simulink model "model"  (R2023b)
settings: Solver=VariableStepAuto  StartTime=0.0  StopTime=10.0  RelTol=1e-3
undefined symbols (not defined in the file): DiscIntNeverNeededParam, fd74c4e2, magnitude, Newton, Raphson
libraries: simulink x102, slpidlib x35
(part 3 of 5)

== system model/cfblk53/cfblk10 ==
  cfblk1 : Inport
  cfblk10 : Inport  Port=2
  cfblk11 : Delay  SampleTime=1
  cfblk3 : simulink/Discrete/Tapped Delay  vinit=0.0  samptime=-1  NumDelays=1  DelayOrder=Oldest  includeCurrent=off
  cfblk4 : slpidlib/PID Controller  Controller=PID  Form=Parallel  TimeDomain=Discrete-time  UseExternalTs=off  SampleTime=1  IntegratorMethod=Forward Euler  FilterMethod=Forward Euler  ControllerParametersSource=internal  P=1  I=1  UseKiTs=off  D=0  N=100  UseFilter=on  TunerSelectOption=Transfer Function Based (PID Tuner App)  InitialConditionSource=internal  InitialConditionForIntegrator=0  InitialConditionForFilter=0  DifferentiatorICPrevScaledInput=0  ExternalReset=none  TrackingMode=off  Kt=1  LimitOutput=off  SatLimitsSource=internal  UpperSaturationLimit=inf  LowerSaturationLimit=-inf  LinearizeAsGain=off  AntiWindupMode=none  Kb=1  LimitIntegrator=off  UpperIntegratorSaturationLimit=inf  LowerIntegratorSaturationLimit=-inf  POutMin=[]  POutMax=[]  IOutMin=[]  IOutMax=[]  DOutMin=[]  DOutMax=[]  NOutMin=[]  NOutMax=[]  SumOutMin=[]  SumOutMax=[]  SaturationOutMin=[]  SaturationOutMax=[]  PParamMin=[]  PParamMax=[]  IParamMin=[]  IParamMax=[]  DParamMin=[]  DParamMax=[]  NParamMin=[]  NParamMax=[]  KbParamMin=[]  KbParamMax=[]  KtParamMin=[]  KtParamMax=[]  KbOutMin=[]  KbOutMax=[]  KtOutMin=[]  KtOutMax=[]  IntegratorOutMin=[]  IntegratorOutMax=[]  FilterOutMin=[]  FilterOutMax=[]  SumI1OutMin=[]  SumI1OutMax=[]  SumI2OutMin=[]  SumI2OutMax=[]  SumI3OutMin=[]  SumI3OutMax=[]  SumI4OutMin=[]  SumI4OutMax=[]  SumDOutMin=[]  SumDOutMax=[]  DifferentiatorOutMin=[]  DifferentiatorOutMax=[]  FilterDiffOutCoefMin=[]  FilterDiffOutCoefMax=[]  ReciprocalOutMin=[]  ReciprocalOutMax=[]  SumDenOutMin=[]  SumDenOutMax=[]  SumNumOutMin=[]  SumNumOutMax=[]  DivideOutMin=[]  DivideOutMax=[]  UdiffTsProdOutMin=[]  UdiffTsProdOutMax=[]  NTsProdOutMin=[]  NTsProdOutMax=[]  UintegralTsProdOutMin=[]  UintegralTsProdOutMax=[]  UngainTsProdOutMin=[]  UngainTsProdOutMax=[]  ClampingZeroOutDataTypeStr=Inherit: Inherit via back propagation  ClampingZeroOutMin=[]  ClampingZeroOutMax=[]  FilterDenConstantOutDataTypeStr=Inherit: Inherit via back propagation  FilterDenConstantOutMin=[]  FilterDenConstantOutMax=[]  PCopyOutDataTypeStr=Inherit: Inherit via back propagation  PCopyOutMin=[]  PCopyOutMax=[]  NCopyOutDataTypeStr=Inherit: Inherit via back propagation  NCopyOutMin=[]  NCopyOutMax=[]  IntegratorContinuousStateAttributes=''  IntegratorStateMustResolveToSignalObject=off  IntegratorRTWStateStorageClass=Auto  FilterContinuousStateAttributes=''  FilterStateMustResolveToSignalObject=off  FilterRTWStateStorageClass=Auto  ParallelPVariant=InternalParameters  IdealPVariant=Disabled  IVariant=InternalParameters  DVariant=InternalParameters  IntegratorVariant=Discrete  SatVariant=Disabled  AWVariant=Passthrough  PCopyVariant=Disabled  TRVariant=Disabled  FdbkBlocksVariant=Forward  IdealPFdbkVariant=Disabled  SatFdbkVariant=Disabled  DerivativeFilterVariant=ForwardEulerFilter  NVariant=InternalParameters  NCopyVariant=Disabled  FilterICVariant=InternalICsFilter  IntegratorICVariant=InternalICs  ExternalResetVariant=Disabled  TRSumVariant=Passthrough  SumFdbkVariant=Disabled  SumVariant=Sum_PID  TsampFilterVariant=InternalTs  TsampNgainVariant=Passthrough  TsampIntegralVariant=Disabled_SignalSpec  ExternalSaturationOutDataTypeStr=Inherit: Same as second input
      settings: LibrarySourceBlock=simulink/Discrete/Discrete PID Controller
  cfblk5 : DiscreteIntegrator  ICPrevOutput=DiscIntNeverNeededParam  ICPrevScaledInput=DiscIntNeverNeededParam
  cfblk6 : Reshape
  cfblk7 : Sum  Inputs=+-
  cfblk8 : Gain  Gain=[817664659.316137]
  cfblk9 : ComplexToMagnitudeAngle
  cfblk2 : Outport
  wires:
  cfblk7/1 -> cfblk2/1
  cfblk1/1 -> cfblk7/1
  cfblk4/1 -> cfblk6/1
  cfblk8/1 -> cfblk9/1
  cfblk9/1 -> cfblk3/1
  cfblk3/1 -> cfblk5/1
  cfblk10/1 -> cfblk8/1
  cfblk9/2 -> cfblk7/2
  cfblk6/1 -> cfblk11/1
  cfblk11/1 -> cfblk4/1

== system model/cfblk53/cfblk11 ==
  cfblk1 : Inport
  cfblk7 : Inport  Port=2
  cfblk8 : Inport  Port=3
  cfblk9 : Inport  Port=4
  cfblk3 : simulink/Discrete/Transfer Fcn Lead or Lag  PoleZ=0.95  ZeroZ=0.75  ICPrevOutput=0.0  ICPrevInput=0.0  DoSatur=off
  cfblk4 : simulink/Discrete/Difference  ICPrevInput=0.0  OutMin=[]  OutMax=[]  OutDataTypeStr=Inherit: Inherit via back propagation  OutDataType=fixdt(1, 16)  OutScaling=2^-10  DoSatur=off
  cfblk5 : Product  Inputs=*
  cfblk6 : Sum  Inputs=+
  cfblk2 : Outport
  cfblk10 : Outport  Port=2
  cfblk11 : Outport  Port=3
  wires:
  cfblk5/1 -> cfblk2/1
  cfblk3/1 -> cfblk10/1
  cfblk6/1 -> cfblk11/1
  cfblk1/1 -> cfblk3/1
  cfblk8/1 -> cfblk6/1
  cfblk4/1 -> cfblk5/1
  cfblk7/1 -> cfblk4/1

== system model/cfblk53/cfblk12 ==
  cfblk1 : Inport
  cfblk13 : Inport  Port=2
  cfblk14 : Inport  Port=3
  cfblk10 : Constant  Value=[-206110537.418355]  SampleTime=1
  cfblk11 : Constant  Value=[146359783.021186]  SampleTime=1
  cfblk12 : Constant  Value=[-708907228.749983]  SampleTime=1
  cfblk3 : DiscreteZeroPole  Poles=[0 0.5]  Gain=1
  cfblk4 : DiscreteFilter  SampleTime=1
  cfblk5 : Delay  DelayLengthSource=Input port  SampleTime=1
      settings: InputPortMap=u0,p1
  cfblk6 : DiscreteStateSpace
  cfblk7 : Abs  SaturateOnIntegerOverflow=off
  cfblk8 : Product
  cfblk9 : Sin  TimeSource=Use external signal  SampleTime=0
  cfblk2 : Outport
  wires:
  cfblk3/1 -> cfblk6/1
  cfblk10/1 -> cfblk4/1
  cfblk7/1 -> cfblk8/1
  cfblk12/1 -> cfblk8/2
  cfblk9/1 -> cfblk2/1
  cfblk6/1 -> cfblk9/1
  cfblk8/1 -> cfblk5/1
  cfblk13/1 -> cfblk3/1
  cfblk1/1 -> cfblk7/1
  cfblk14/1 -> cfblk5/2

== system model/cfblk55/cfblk10 ==
  cfblk1 : Inport
  cfblk12 : Inport  Port=2
  cfblk13 : Inport  Port=3
  cfblk14 : Inport  Port=4
  cfblk10 : Constant  Value=[62866536.244015]  SampleTime=1
  cfblk11 : Constant  Value=[-503289504.904032]  SampleTime=1
  cfblk3 : slpidlib/PID Controller (2DOF)  Controller=PID  Form=Parallel  TimeDomain=Discrete-time  UseExternalTs=off  SampleTime=1  IntegratorMethod=Forward Euler  FilterMethod=Forward Euler  ControllerParametersSource=internal  P=1  I=1  UseKiTs=off  D=0  N=100  UseFilter=on  b=1  c=1  TunerSelectOption=Transfer Function Based (PID Tuner App)  InitialConditionSource=internal  InitialConditionForIntegrator=0  InitialConditionForFilter=0  DifferentiatorICPrevScaledInput=0  ExternalReset=none  TrackingMode=off  Kt=1  LimitOutput=off  SatLimitsSource=internal  UpperSaturationLimit=inf  LowerSaturationLimit=-inf  LinearizeAsGain=off  AntiWindupMode=none  Kb=1  LimitIntegrator=off  UpperIntegratorSaturationLimit=inf  LowerIntegratorSaturationLimit=-inf  POutMin=[]  POutMax=[]  IOutMin=[]  IOutMax=[]  DOutMin=[]  DOutMax=[]  NOutMin=[]  NOutMax=[]  bOutMin=[]  bOutMax=[]  cOutMin=[]  cOutMax=[]  SumOutMin=[]  SumOutMax=[]  SaturationOutMin=[]  SaturationOutMax=[]  PParamMin=[]  PParamMax=[]  IParamMin=[]  IParamMax=[]  DParamMin=[]  DParamMax=[]  NParamMin=[]  NParamMax=[]  bParamMin=[]  bParamMax=[]  cParamMin=[]  cParamMax=[]  KbParamMin=[]  KbParamMax=[]  KtParamMin=[]  KtParamMax=[]  KbOutMin=[]  KbOutMax=[]  KtOutMin=[]  KtOutMax=[]  IntegratorOutMin=[]  IntegratorOutMax=[]  FilterOutMin=[]  FilterOutMax=[]  SumI1OutMin=[]  SumI1OutMax=[]  SumI2OutMin=[]  SumI2OutMax=[]  SumI3OutMin=[]  SumI3OutMax=[]  SumI4OutMin=[]  SumI4OutMax=[]  SumDOutMin=[]  SumDOutMax=[]  Sum1OutMin=[]  Sum1OutMax=[]  Sum2OutMin=[]  Sum2OutMax=[]  Sum3OutMin=[]  Sum3OutMax=[]  DifferentiatorOutMin=[]  DifferentiatorOutMax=[]  FilterDiffOutCoefMin=[]  FilterDiffOutCoefMax=[]  ReciprocalOutMin=[]  ReciprocalOutMax=[]  SumDenOutMin=[]  SumDenOutMax=[]  SumNumOutMin=[]  SumNumOutMax=[]  DivideOutMin=[]  DivideOutMax=[]  UdiffTsProdOutMin=[]  UdiffTsProdOutMax=[]  NTsProdOutMin=[]  NTsProdOutMax=[]  UintegralTsProdOutMin=[]  UintegralTsProdOutMax=[]  UngainTsProdOutMin=[]  UngainTsProdOutMax=[]  ClampingZeroOutDataTypeStr=Inherit: Inherit via back propagation  ClampingZeroOutMin=[]  ClampingZeroOutMax=[]  FilterDenConstantOutDataTypeStr=Inherit: Inherit via back propagation  FilterDenConstantOutMin=[]  FilterDenConstantOutMax=[]  PCopyOutDataTypeStr=Inherit: Inherit via back propagation  PCopyOutMin=[]  PCopyOutMax=[]  NCopyOutDataTypeStr=Inherit: Inherit via back propagation  NCopyOutMin=[]  NCopyOutMax=[]  IntegratorContinuousStateAttributes=''  IntegratorStateMustResolveToSignalObject=off  IntegratorRTWStateStorageClass=Auto  FilterContinuousStateAttributes=''  FilterStateMustResolveToSignalObject=off  FilterRTWStateStorageClass=Auto  ParallelPVariant=InternalParameters  IdealPVariant=Disabled  IVariant=InternalParameters  DVariant=InternalParameters  bVariant=InternalParameters  cVariant=InternalParameters  IntegratorVariant=Discrete  SatVariant=Disabled  AWVariant=Passthrough  PCopyVariant=Disabled  TRVariant=Disabled  FdbkBlocksVariant=Forward  IdealPFdbkVariant=Disabled  SatFdbkVariant=Disabled  DerivativeFilterVariant=ForwardEulerFilter  NVariant=InternalParameters  NCopyVariant=Disabled  FilterICVariant=InternalICsFilter  IntegratorICVariant=InternalICs  ExternalResetVariant=Disabled  TRSumVariant=Passthrough  SumFdbkVariant=Disabled  SumVariant=Sum_PID  TsampFilterVariant=InternalTs  TsampNgainVariant=Passthrough  TsampIntegralVariant=Disabled_SignalSpec  ExternalSaturationOutDataTypeStr=Inherit: Same as second input
      settings: LibrarySourceBlock=simulink/Discrete/Discrete PID Controller (2DOF)
  cfblk4 : slpidlib/PID Controller (2DOF)  Controller=PID  Form=Parallel  TimeDomain=Discrete-time  UseExternalTs=off  SampleTime=1  IntegratorMethod=Forward Euler  FilterMethod=Forward Euler  ControllerParametersSource=internal  P=1  I=1  UseKiTs=off  D=0  N=100  UseFilter=on  b=1  c=1  TunerSelectOption=Transfer Function Based (PID Tuner App)  InitialConditionSource=internal  InitialConditionForIntegrator=0  InitialConditionForFilter=0  DifferentiatorICPrevScaledInput=0  ExternalReset=none  TrackingMode=off  Kt=1  LimitOutput=off  SatLimitsSource=internal  UpperSaturationLimit=inf  LowerSaturationLimit=-inf  LinearizeAsGain=off  AntiWindupMode=none  Kb=1  LimitIntegrator=off  UpperIntegratorSaturationLimit=inf  LowerIntegratorSaturationLimit=-inf  POutMin=[]  POutMax=[]  IOutMin=[]  IOutMax=[]  DOutMin=[]  DOutMax=[]  NOutMin=[]  NOutMax=[]  bOutMin=[]  bOutMax=[]  cOutMin=[]  cOutMax=[]  SumOutMin=[]  SumOutMax=[]  SaturationOutMin=[]  SaturationOutMax=[]  PParamMin=[]  PParamMax=[]  IParamMin=[]  IParamMax=[]  DParamMin=[]  DParamMax=[]  NParamMin=[]  NParamMax=[]  bParamMin=[]  bParamMax=[]  cParamMin=[]  cParamMax=[]  KbParamMin=[]  KbParamMax=[]  KtParamMin=[]  KtParamMax=[]  KbOutMin=[]  KbOutMax=[]  KtOutMin=[]  KtOutMax=[]  IntegratorOutMin=[]  IntegratorOutMax=[]  FilterOutMin=[]  FilterOutMax=[]  SumI1OutMin=[]  SumI1OutMax=[]  SumI2OutMin=[]  SumI2OutMax=[]  SumI3OutMin=[]  SumI3OutMax=[]  SumI4OutMin=[]  SumI4OutMax=[]  SumDOutMin=[]  SumDOutMax=[]  Sum1OutMin=[]  Sum1OutMax=[]  Sum2OutMin=[]  Sum2OutMax=[]  Sum3OutMin=[]  Sum3OutMax=[]  DifferentiatorOutMin=[]  DifferentiatorOutMax=[]  FilterDiffOutCoefMin=[]  FilterDiffOutCoefMax=[]  ReciprocalOutMin=[]  ReciprocalOutMax=[]  SumDenOutMin=[]  SumDenOutMax=[]  SumNumOutMin=[]  SumNumOutMax=[]  DivideOutMin=[]  DivideOutMax=[]  UdiffTsProdOutMin=[]  UdiffTsProdOutMax=[]  NTsProdOutMin=[]  NTsProdOutMax=[]  UintegralTsProdOutMin=[]  UintegralTsProdOutMax=[]  UngainTsProdOutMin=[]  UngainTsProdOutMax=[]  ClampingZeroOutDataTypeStr=Inherit: Inherit via back propagation  ClampingZeroOutMin=[]  ClampingZeroOutMax=[]  FilterDenConstantOutDataTypeStr=Inherit: Inherit via back propagation  FilterDenConstantOutMin=[]  FilterDenConstantOutMax=[]  PCopyOutDataTypeStr=Inherit: Inherit via back propagation  PCopyOutMin=[]  PCopyOutMax=[]  NCopyOutDataTypeStr=Inherit: Inherit via back propagation  NCopyOutMin=[]  NCopyOutMax=[]  IntegratorContinuousStateAttributes=''  IntegratorStateMustResolveToSignalObject=off  IntegratorRTWStateStorageClass=Auto  FilterContinuousStateAttributes=''  FilterStateMustResolveToSignalObject=off  FilterRTWStateStorageClass=Auto  ParallelPVariant=InternalParameters  IdealPVariant=Disabled  IVariant=InternalParameters  DVariant=InternalParameters  bVariant=InternalParameters  cVariant=InternalParameters  IntegratorVariant=Discrete  SatVariant=Disabled  AWVariant=Passthrough  PCopyVariant=Disabled  TRVariant=Disabled  FdbkBlocksVariant=Forward  IdealPFdbkVariant=Disabled  SatFdbkVariant=Disabled  DerivativeFilterVariant=ForwardEulerFilter  NVariant=InternalParameters  NCopyVariant=Disabled  FilterICVariant=InternalICsFilter  IntegratorICVariant=InternalICs  ExternalResetVariant=Disabled  TRSumVariant=Passthrough  SumFdbkVariant=Disabled  SumVariant=Sum_PID  TsampFilterVariant=InternalTs  TsampNgainVariant=Passthrough  TsampIntegralVariant=Disabled_SignalSpec  ExternalSaturationOutDataTypeStr=Inherit: Same as second input
      settings: LibrarySourceBlock=simulink/Discrete/Discrete PID Controller (2DOF)
  cfblk5 : DiscreteStateSpace
  cfblk6 : Bias  Bias=[716171832.572191]  SaturateOnIntegerOverflow=off
  cfblk7 : Polyval  Coefs=[ +2.081618890e-019, -1.441693666e-014, +4.719686976e-010, -8.536869453e-006, +1.621573104e-001, -8.087801117e+001 ]
  cfblk8 : Constant  Value=[-316048415.208695]  SampleTime=1
  cfblk9 : Constant  Value=[-244945707.494813]  SampleTime=1
  cfblk2 : Outport
  cfblk15 : Outport  Port=2
  wires:
  cfblk6/1 -> cfblk5/1
  cfblk5/1 -> cfblk3/1
  cfblk1/1 -> cfblk4/1
  cfblk9/1 -> cfblk4/2
  cfblk8/1 -> cfblk3/2
  cfblk3/1 -> cfblk7/1
  cfblk10/1 -> cfblk15/1
  cfblk12/1 -> cfblk2/1
  cfblk13/1 -> cfblk6/1

== system model/cfblk55/cfblk11 ==
  cfblk1 : Inport
  cfblk9 : Inport  Port=2
  cfblk10 : Inport  Port=3
  cfblk11 : Inport  Port=4
  cfblk12 : Inport  Port=5
  cfblk13 : Inport  Port=6
  cfblk3 : DiscreteIntegrator  ICPrevOutput=DiscIntNeverNeededParam  ICPrevScaledInput=DiscIntNeverNeededParam
  cfblk4 : DiscreteStateSpace
  cfblk5 : ComplexToRealImag
  cfblk6 : Sum  Inputs=+-
  cfblk7 : Constant  Value=[-907148050.764415]  SampleTime=1
  cfblk8 : Constant  Value=[-534592741.405864]  SampleTime=1
  cfblk2 : Outport
  cfblk14 : Outport  Port=2
  wires:
  cfblk3/1 -> cfblk5/1
  cfblk1/1 -> cfblk14/1
  cfblk6/1 -> cfblk2/1
  cfblk8/1 -> cfblk6/1
  cfblk12/1 -> cfblk3/1
  cfblk11/1 -> cfblk4/1
  cfblk10/1 -> cfblk6/2

== system model/cfblk55/cfblk12 ==
  cfblk1 : Inport
  cfblk10 : Inport  Port=2
  cfblk11 : Inport  Port=3
  cfblk3 : simulink/Discrete/Transfer Fcn First Order  PoleZ=0.95  ICPrevOutput=0.0  DoSatur=off
  cfblk4 : UnitDelay  HasFrameUpgradeWarning=on
  cfblk5 : DiscreteFilter  SampleTime=1
  cfblk6 : simulink/Discrete/Difference  ICPrevInput=0.0  OutMin=[]  OutMax=[]  OutDataTypeStr=Inherit: Inherit via back propagation  OutDataType=fixdt(1, 16)  OutScaling=2^-10  DoSatur=off
  cfblk7 : Sqrt  Operator=rSqrt  AlgorithmType=Newton-Raphson
  cfblk8 : Product  Inputs=*
  cfblk9 : Constant  Value=[-99960536.236063]  SampleTime=1
  cfblk2 : Outport
  cfblk12 : Outport  Port=2
  wires:
  cfblk11/1 -> cfblk8/1
  cfblk9/1 -> cfblk3/1
  cfblk1/1 -> cfblk12/1
  cfblk8/1 -> cfblk5/1
  cfblk10/1 -> cfblk6/1
  cfblk6/1 -> cfblk4/1
  cfblk5/1 -> cfblk2/1
  cfblk4/1 -> cfblk7/1

== system model/cfblk56/cfblk10 ==
  cfblk1 : Inport
  cfblk7 : Inport  Port=2
  cfblk8 : Inport  Port=3
  cfblk3 : slpidlib/PID Controller (2DOF)  Controller=PID  Form=Parallel  TimeDomain=Discrete-time  UseExternalTs=off  SampleTime=1  IntegratorMethod=Forward Euler  FilterMethod=Forward Euler  ControllerParametersSource=internal  P=1  I=1  UseKiTs=off  D=0  N=100  UseFilter=on  b=1  c=1  TunerSelectOption=Transfer Function Based (PID Tuner App)  InitialConditionSource=internal  InitialConditionForIntegrator=0  InitialConditionForFilter=0  DifferentiatorICPrevScaledInput=0  ExternalReset=none  TrackingMode=off  Kt=1  LimitOutput=off  SatLimitsSource=internal  UpperSaturationLimit=inf  LowerSaturationLimit=-inf  LinearizeAsGain=off  AntiWindupMode=none  Kb=1  LimitIntegrator=off  UpperIntegratorSaturationLimit=inf  LowerIntegratorSaturationLimit=-inf  POutMin=[]  POutMax=[]  IOutMin=[]  IOutMax=[]  DOutMin=[]  DOutMax=[]  NOutMin=[]  NOutMax=[]  bOutMin=[]  bOutMax=[]  cOutMin=[]  cOutMax=[]  SumOutMin=[]  SumOutMax=[]  SaturationOutMin=[]  SaturationOutMax=[]  PParamMin=[]  PParamMax=[]  IParamMin=[]  IParamMax=[]  DParamMin=[]  DParamMax=[]  NParamMin=[]  NParamMax=[]  bParamMin=[]  bParamMax=[]  cParamMin=[]  cParamMax=[]  KbParamMin=[]  KbParamMax=[]  KtParamMin=[]  KtParamMax=[]  KbOutMin=[]  KbOutMax=[]  KtOutMin=[]  KtOutMax=[]  IntegratorOutMin=[]  IntegratorOutMax=[]  FilterOutMin=[]  FilterOutMax=[]  SumI1OutMin=[]  SumI1OutMax=[]  SumI2OutMin=[]  SumI2OutMax=[]  SumI3OutMin=[]  SumI3OutMax=[]  SumI4OutMin=[]  SumI4OutMax=[]  SumDOutMin=[]  SumDOutMax=[]  Sum1OutMin=[]  Sum1OutMax=[]  Sum2OutMin=[]  Sum2OutMax=[]  Sum3OutMin=[]  Sum3OutMax=[]  DifferentiatorOutMin=[]  DifferentiatorOutMax=[]  FilterDiffOutCoefMin=[]  FilterDiffOutCoefMax=[]  ReciprocalOutMin=[]  ReciprocalOutMax=[]  SumDenOutMin=[]  SumDenOutMax=[]  SumNumOutMin=[]  SumNumOutMax=[]  DivideOutMin=[]  DivideOutMax=[]  UdiffTsProdOutMin=[]  UdiffTsProdOutMax=[]  NTsProdOutMin=[]  NTsProdOutMax=[]  UintegralTsProdOutMin=[]  UintegralTsProdOutMax=[]  UngainTsProdOutMin=[]  UngainTsProdOutMax=[]  ClampingZeroOutDataTypeStr=Inherit: Inherit via back propagation  ClampingZeroOutMin=[]  ClampingZeroOutMax=[]  FilterDenConstantOutDataTypeStr=Inherit: Inherit via back propagation  FilterDenConstantOutMin=[]  FilterDenConstantOutMax=[]  PCopyOutDataTypeStr=Inherit: Inherit via back propagation  PCopyOutMin=[]  PCopyOutMax=[]  NCopyOutDataTypeStr=Inherit: Inherit via back propagation  NCopyOutMin=[]  NCopyOutMax=[]  IntegratorContinuousStateAttributes=''  IntegratorStateMustResolveToSignalObject=off  IntegratorRTWStateStorageClass=Auto  FilterContinuousStateAttributes=''  FilterStateMustResolveToSignalObject=off  FilterRTWStateStorageClass=Auto  ParallelPVariant=InternalParameters  IdealPVariant=Disabled  IVariant=InternalParameters  DVariant=InternalParameters  bVariant=InternalParameters  cVariant=InternalParameters  IntegratorVariant=Discrete  SatVariant=Disabled  AWVariant=Passthrough  PCopyVariant=Disabled  TRVariant=Disabled  FdbkBlocksVariant=Forward  IdealPFdbkVariant=Disabled  SatFdbkVariant=Disabled  DerivativeFilterVariant=ForwardEulerFilter  NVariant=InternalParameters  NCopyVariant=Disabled  FilterICVariant=InternalICsFilter  IntegratorICVariant=InternalICs  ExternalResetVariant=Disabled  TRSumVariant=Passthrough  SumFdbkVariant=Disabled  SumVariant=Sum_PID  TsampFilterVariant=InternalTs  TsampNgainVariant=Passthrough  TsampIntegralVariant=Disabled_SignalSpec  ExternalSaturationOutDataTypeStr=Inherit: Same as second input
      settings: LibrarySourceBlock=simulink/Discrete/Discrete PID Controller (2DOF)
  cfblk4 : UnitDelay  HasFrameUpgradeWarning=on
  cfblk5 : Sum  Inputs=|++
  cfblk6 : Constant  Value=[238161713.351589]  SampleTime=1
  cfblk2 : Outport
  wires:
  cfblk3/1 -> cfblk2/1
  cfblk1/1 -> cfblk3/1
  cfblk6/1 -> cfblk4/1
  cfblk7/1 -> cfblk5/1
  cfblk4/1 -> cfblk3/2
  cfblk8/1 -> cfblk5/2

== system model/cfblk56/cfblk8 ==
  cfblk1 : Inport
  cfblk10 : Delay  SampleTime=1
  cfblk3 : DiscreteFir  SampleTime=1
  cfblk4 : simulink/Discrete/Tapped Delay  vinit=0.0  samptime=-1  NumDelays=1  DelayOrder=Oldest  includeCurrent=off
  cfblk5 : slpidlib/PID Controller (2DOF)  Controller=PID  Form=Parallel  TimeDomain=Discrete-time  UseExternalTs=off  SampleTime=1  IntegratorMethod=Forward Euler  FilterMethod=Forward Euler  ControllerParametersSource=internal  P=1  I=1  UseKiTs=off  D=0  N=100  UseFilter=on  b=1  c=1  TunerSelectOption=Transfer Function Based (PID Tuner App)  InitialConditionSource=internal  InitialConditionForIntegrator=0  InitialConditionForFilter=0  DifferentiatorICPrevScaledInput=0  ExternalReset=none  TrackingMode=off  Kt=1  LimitOutput=off  SatLimitsSource=internal  UpperSaturationLimit=inf  LowerSaturationLimit=-inf  LinearizeAsGain=off  AntiWindupMode=none  Kb=1  LimitIntegrator=off  UpperIntegratorSaturationLimit=inf  LowerIntegratorSaturationLimit=-inf  POutMin=[]  POutMax=[]  IOutMin=[]  IOutMax=[]  DOutMin=[]  DOutMax=[]  NOutMin=[]  NOutMax=[]  bOutMin=[]  bOutMax=[]  cOutMin=[]  cOutMax=[]  SumOutMin=[]  SumOutMax=[]  SaturationOutMin=[]  SaturationOutMax=[]  PParamMin=[]  PParamMax=[]  IParamMin=[]  IParamMax=[]  DParamMin=[]  DParamMax=[]  NParamMin=[]  NParamMax=[]  bParamMin=[]  bParamMax=[]  cParamMin=[]  cParamMax=[]  KbParamMin=[]  KbParamMax=[]  KtParamMin=[]  KtParamMax=[]  KbOutMin=[]  KbOutMax=[]  KtOutMin=[]  KtOutMax=[]  IntegratorOutMin=[]  IntegratorOutMax=[]  FilterOutMin=[]  FilterOutMax=[]  SumI1OutMin=[]  SumI1OutMax=[]  SumI2OutMin=[]  SumI2OutMax=[]  SumI3OutMin=[]  SumI3OutMax=[]  SumI4OutMin=[]  SumI4OutMax=[]  SumDOutMin=[]  SumDOutMax=[]  Sum1OutMin=[]  Sum1OutMax=[]  Sum2OutMin=[]  Sum2OutMax=[]  Sum3OutMin=[]  Sum3OutMax=[]  DifferentiatorOutMin=[]  DifferentiatorOutMax=[]  FilterDiffOutCoefMin=[]  FilterDiffOutCoefMax=[]  ReciprocalOutMin=[]  ReciprocalOutMax=[]  SumDenOutMin=[]  SumDenOutMax=[]  SumNumOutMin=[]  SumNumOutMax=[]  DivideOutMin=[]  DivideOutMax=[]  UdiffTsProdOutMin=[]  UdiffTsProdOutMax=[]  NTsProdOutMin=[]  NTsProdOutMax=[]  UintegralTsProdOutMin=[]  UintegralTsProdOutMax=[]  UngainTsProdOutMin=[]  UngainTsProdOutMax=[]  ClampingZeroOutDataTypeStr=Inherit: Inherit via back propagation  ClampingZeroOutMin=[]  ClampingZeroOutMax=[]  FilterDenConstantOutDataTypeStr=Inherit: Inherit via back propagation  FilterDenConstantOutMin=[]  FilterDenConstantOutMax=[]  PCopyOutDataTypeStr=Inherit: Inherit via back propagation  PCopyOutMin=[]  PCopyOutMax=[]  NCopyOutDataTypeStr=Inherit: Inherit via back propagation  NCopyOutMin=[]  NCopyOutMax=[]  IntegratorContinuousStateAttributes=''  IntegratorStateMustResolveToSignalObject=off  IntegratorRTWStateStorageClass=Auto  FilterContinuousStateAttributes=''  FilterStateMustResolveToSignalObject=off  FilterRTWStateStorageClass=Auto  ParallelPVariant=InternalParameters  IdealPVariant=Disabled  IVariant=InternalParameters  DVariant=InternalParameters  bVariant=InternalParameters  cVariant=InternalParameters  IntegratorVariant=Discrete  SatVariant=Disabled  AWVariant=Passthrough  PCopyVariant=Disabled  TRVariant=Disabled  FdbkBlocksVariant=Forward  IdealPFdbkVariant=Disabled  SatFdbkVariant=Disabled  DerivativeFilterVariant=ForwardEulerFilter  NVariant=InternalParameters  NCopyVariant=Disabled  FilterICVariant=InternalICsFilter  IntegratorICVariant=InternalICs  ExternalResetVariant=Disabled  TRSumVariant=Passthrough  SumFdbkVariant=Disabled  SumVariant=Sum_PID  TsampFilterVariant=InternalTs  TsampNgainVariant=Passthrough  TsampIntegralVariant=Disabled_SignalSpec  ExternalSaturationOutDataTypeStr=Inherit: Same as second input
      settings: LibrarySourceBlock=simulink/Discrete/Discrete PID Controller (2DOF)
  cfblk6 : Trigonometry
  cfblk7 : Sqrt
  cfblk8 : Constant  Value=[-876494320.439863]  SampleTime=1
  cfblk2 : Outport
  cfblk9 : Outport  Port=2
  wires:
  cfblk8/1 -> cfblk6/1
  cfblk3/1 -> cfblk5/1
  cfblk5/1 -> cfblk2/1, cfblk7/1
  cfblk7/1 -> cfblk4/1
  cfblk1/1 -> cfblk9/1
  cfblk6/1 -> cfblk5/2
  cfblk4/1 -> cfblk10/1
  cfblk10/1 -> cfblk3/1

== system model/cfblk56/cfblk9 ==
  cfblk1 : Inport
  cfblk7 : Inport  Port=2
  cfblk3 : Gain  Gain=[-414813856.337877]
  cfblk4 : Polyval  Coefs=[ +2.081618890e-019, -1.441693666e-014, +4.719686976e-010, -8.536869453e-006, +1.621573104e-001, -8.087801117e+001 ]
  cfblk5 : Product  Inputs=**
  cfblk6 : Constant  Value=[863840026.275100]  SampleTime=1
  cfblk2 : Outport
  cfblk8 : Outport  Port=2
  wires:
  cfblk7/1 -> cfblk3/1
  cfblk6/1 -> cfblk5/1
  cfblk1/1 -> cfblk5/2
  cfblk5/1 -> cfblk8/1
  cfblk4/1 -> cfblk2/1
  cfblk3/1 -> cfblk4/1

== system model/cfblk57/cfblk10 ==
  cfblk1 : Inport
  cfblk15 : Inport  Port=2
  cfblk16 : Inport  Port=3
  cfblk10 : Sum  Inputs=+-
  cfblk11 : Product  Inputs=*
  cfblk12 : Constant  Value=[214957307.800664]  SampleTime=1
  cfblk13 : Constant  Value=[-547301041.829441]  SampleTime=1
  cfblk14 : Constant  Value=[871990443.068065]  SampleTime=1
  cfblk18 : Delay  SampleTime=1
  cfblk3 : simulink/Discrete/Tapped Delay  vinit=0.0  samptime=-1  NumDelays=1  DelayOrder=Oldest  includeCurrent=off
  cfblk4 : DiscreteZeroPole  Poles=[0 0.5]  Gain=1
  cfblk5 : DiscreteIntegrator  ICPrevOutput=DiscIntNeverNeededParam  ICPrevScaledInput=DiscIntNeverNeededParam
  cfblk6 : simulink/Math Operations/Slider Gain  gain=1  low=0  high=2
  cfblk7 : Gain  Gain=[-961031888.110048]
  cfblk8 : Sum  Inputs=+-
  cfblk9 : Signum
  cfblk2 : Outport
  cfblk17 : Outport  Port=2
  wires:
  cfblk10/1 -> cfblk9/1
  cfblk1/1 -> cfblk4/1
  cfblk12/1 -> cfblk5/1
  cfblk6/1 -> cfblk3/1
  cfblk11/1 -> cfblk17/1
  cfblk3/1 -> cfblk8/1
  cfblk15/1 -> cfblk6/1
  cfblk4/1 -> cfblk10/1
  cfblk5/1 -> cfblk11/1
  cfblk13/1 -> cfblk8/2
  cfblk8/1 -> cfblk7/1
  cfblk7/1 -> cfblk2/1
  cfblk9/1 -> cfblk18/1
  cfblk18/1 -> cfblk10/2

== system model/cfblk57/cfblk11 ==
  cfblk1 : Inport
  cfblk10 : Inport  Port=2
  cfblk11 : Inport  Port=3
  cfblk12 : Inport  Port=4
  cfblk3 : simulink/Discrete/Tapped Delay  vinit=0.0  samptime=-1  NumDelays=1  DelayOrder=Oldest  includeCurrent=off
  cfblk4 : simulink/Discrete/Transfer Fcn First Order  PoleZ=0.95  ICPrevOutput=0.0  DoSatur=off
  cfblk5 : simulink/Math Operations/Slider Gain  gain=1  low=0  high=2
  cfblk6 : Polyval  Coefs=[ +2.081618890e-019, -1.441693666e-014, +4.719686976e-010, -8.536869453e-006, +1.621573104e-001, -8.087801117e+001 ]
  cfblk7 : ComplexToMagnitudeAngle
  cfblk8 : Sum  Inputs=|++
  cfblk9 : Sum  Inputs=+
  cfblk2 : Outport
  cfblk13 : Outport  Port=2
  cfblk14 : Outport  Port=3
  wires:
  cfblk3/1 -> cfblk4/1
  cfblk7/1 -> cfblk5/1
  cfblk5/1 -> cfblk3/1
  cfblk1/1 -> cfblk8/1
  cfblk10/1 -> cfblk7/1
  cfblk9/1 -> cfblk14/1
  cfblk12/1 -> cfblk8/2
  cfblk7/2 -> cfblk6/1
  cfblk8/1 -> cfblk2/1
  cfblk4/1 -> cfblk9/1
  cfblk11/1 -> cfblk13/1

== system model/cfblk57/cfblk12 ==
  cfblk1 : Inport
  cfblk13 : Inport  Port=2
  cfblk14 : Inport  Port=3
  cfblk15 : Inport  Port=4
  cfblk10 : Trigonometry
  cfblk11 : Constant  Value=[343190299.712040]  SampleTime=1
  cfblk12 : Constant  Value=[949619341.202744]  SampleTime=1
  cfblk3 : DiscreteZeroPole  Poles=[0 0.5]  Gain=1
  cfblk4 : simulink/Discrete/Transfer Fcn Real Zero  ZeroZ=0.75  ICPrevInput=0.0  DoSatur=off
  cfblk5 : DiscreteTransferFcn  SampleTime=1
  cfblk6 : Sin  TimeSource=Use external signal  SampleTime=0
  cfblk7 : Sum
  cfblk8 : Rounding
  cfblk9 : ComplexToRealImag
  cfblk2 : Outport
  cfblk16 : Outport  Port=2
  cfblk17 : Outport  Port=3
  wires:
  cfblk11/1 -> cfblk7/1
  cfblk1/1 -> cfblk6/1
  cfblk5/1 -> cfblk9/1
  cfblk7/1 -> cfblk8/1
  cfblk14/1 -> cfblk16/1
  cfblk12/1 -> cfblk10/1
  cfblk10/1 -> cfblk4/1
  cfblk6/1 -> cfblk2/1
  cfblk8/1 -> cfblk5/1
  cfblk4/1 -> cfblk3/1
  cfblk15/1 -> cfblk17/1
  cfblk3/1 -> cfblk7/2

== system model/cfblk57/cfblk13 ==
  cfblk1 : Inport
  cfblk11 : Inport  Port=2
  cfblk12 : Inport  Port=3
  cfblk13 : Inport  Port=4
  cfblk10 : Constant  Value=[303947422.520252]  SampleTime=1
  cfblk14 : Delay  SampleTime=1
  cfblk3 : Delay  DelayLengthSource=Input port  SampleTime=1
      settings: InputPortMap=u0,p1
  cfblk4 : Sum  Inputs=+-
  cfblk5 : Product  Inputs=**
  cfblk6 : Assignment  DiagnosticForDimensions=Warning  IndexOptions=Index vector (dialog)  Indices=1  OutputSizes=1
  cfblk7 : Reshape
  cfblk8 : Abs  SaturateOnIntegerOverflow=off
  cfblk9 : Math  Operator=log10
  cfblk2 : Outport
  wires:
  cfblk3/1 -> cfblk6/1
  cfblk13/1 -> cfblk5/1
  cfblk1/1 -> cfblk5/2
  cfblk9/1 -> cfblk4/1
  cfblk6/1 -> cfblk8/1
  cfblk10/1 -> cfblk4/2
  cfblk11/1 -> cfblk7/1
  cfblk12/1 -> cfblk2/1
  cfblk7/1 -> cfblk6/2
  cfblk8/1 -> cfblk9/1
  cfblk5/1 -> cfblk3/2
  cfblk4/1 -> cfblk14/1
  cfblk14/1 -> cfblk3/1

== system model/cfblk57/cfblk14 ==
  cfblk1 : Inport
  cfblk10 : Inport  Port=2
  cfblk12 : Delay  SampleTime=1
  cfblk3 : DiscreteFir  SampleTime=1
  cfblk4 : Delay  SampleTime=1
  cfblk5 : simulink/Math Operations/Slider Gain  gain=1  low=0  high=2
  cfblk6 : Product  Inputs=**
  cfblk7 : Product  Inputs=**
  cfblk8 : simulink/Math Operations/Slider Gain  gain=1  low=0  high=2
  cfblk9 : Constant  Value=[-993453400.176832]  SampleTime=1
  cfblk2 : Outport
  cfblk11 : Outport  Port=2
  wires:
  cfblk4/1 -> cfblk3/1
  cfblk3/1 -> cfblk7/1
  cfblk10/1 -> cfblk5/1
  cfblk9/1 -> cfblk2/1
  cfblk6/1 -> cfblk8/1, cfblk7/2
  cfblk1/1 -> cfblk4/1
  cfblk7/1 -> cfblk11/1
  cfblk5/1 -> cfblk6/2
  cfblk8/1 -> cfblk12/1
  cfblk12/1 -> cfblk6/1

== system model/cfblk57/cfblk15 ==
  cfblk1 : Inport
  cfblk15 : Inport  Port=2
  cfblk10 : ComplexToMagnitudeAngle
  cfblk11 : Sin  TimeSource=Use external signal  SampleTime=0
  cfblk12 : PermuteDimensions
  cfblk13 : Constant  Value=[398074408.357430]  SampleTime=1
  cfblk14 : Constant  Value=[-587353639.300088]  SampleTime=1
  cfblk3 : Delay  ShowEnablePort=on  SampleTime=1
      settings: InputPortMap=u0,e6
  cfblk4 : Delay  SampleTime=1
  cfblk5 : Product  Inputs=*
  cfblk6 : Trigonometry
  cfblk7 : Polyval  Coefs=[ +2.081618890e-019, -1.441693666e-014, +4.719686976e-010, -8.536869453e-006, +1.621573104e-001, -8.087801117e+001 ]
  cfblk8 : PermuteDimensions
  cfblk9 : Sqrt
  cfblk2 : Outport
  wires:
  cfblk8/1 -> cfblk6/1
  cfblk15/1 -> cfblk12/1
  cfblk13/1 -> cfblk4/1
  cfblk7/1 -> cfblk8/1
  cfblk12/1 -> cfblk10/1
  cfblk1/1 -> cfblk7/1
  cfblk9/1 -> cfblk3/1
  cfblk4/1 -> cfblk9/1
  cfblk10/1 -> cfblk5/1
  cfblk3/1 -> cfblk2/1
  cfblk10/2 -> cfblk3/2
  cfblk14/1 -> cfblk11/1

== system model/cfblk57/cfblk7 ==
  cfblk1 : Inport
  cfblk11 : Inport  Port=2
  cfblk10 : Constant  Value=[-113188143.412463]  SampleTime=1
  cfblk3 : Delay  DelayLengthSource=Input port  SampleTime=1
      settings: InputPortMap=u0,p1
  cfblk4 : simulink/Discrete/Tapped Delay  vinit=0.0  samptime=-1  NumDelays=1  DelayOrder=Oldest  includeCurrent=off
  cfblk5 : DiscreteFir  SampleTime=1
  cfblk6 : UnaryMinus
  cfblk7 : simulink/Math Operations/Slider Gain  gain=1  low=0  high=2
  cfblk8 : Product
  cfblk9 : Constant  Value=[276723949.793369]  SampleTime=1
  cfblk2 : Outport
  cfblk12 : Outport  Port=2
  cfblk13 : Outport  Port=3
  wires:
  cfblk5/1 -> cfblk12/1
  cfblk8/1 -> cfblk7/1
  cfblk6/1 -> cfblk3/1
  cfblk11/1 -> cfblk2/1
  cfblk9/1 -> cfblk8/1
  cfblk7/1 -> cfblk13/1
  cfblk4/1 -> cfblk5/1
  cfblk3/1 -> cfblk8/2
  cfblk1/1 -> cfblk6/1, cfblk4/1
  cfblk10/1 -> cfblk3/2

== system model/cfblk57/cfblk8 ==
  cfblk1 : Inport
  cfblk8 : Inport  Port=2
  cfblk9 : Inport  Port=3
  cfblk10 : Inport  Port=4
  cfblk11 : Inport  Port=5
  cfblk13 : Delay  SampleTime=1
  cfblk3 : Delay  ShowEnablePort=on  SampleTime=1
      settings: InputPortMap=u0,e6
  cfblk4 : DiscreteFir  SampleTime=1
  cfblk5 : ComplexToRealImag
  cfblk6 : Sum  Inputs=-+
  cfblk7 : ComplexToRealImag
  cfblk2 : Outport
  cfblk12 : Outport  Port=2
  wires:
  cfblk3/1 -> cfblk7/1
  cfblk8/1 -> cfblk12/1
  cfblk10/1 -> cfblk2/1
  cfblk1/1 -> cfblk6/1
  cfblk6/1 -> cfblk4/1
  cfblk9/1 -> cfblk6/2
  cfblk11/1 -> cfblk5/1
  cfblk4/1 -> cfblk3/2
  cfblk7/1 -> cfblk13/1
  cfblk13/1 -> cfblk3/1

== system model/cfblk57/cfblk9 ==
  cfblk1 : Inport
  cfblk12 : Inport  Port=2
  cfblk13 : Inport  Port=3
  cfblk10 : Squeeze
  cfblk11 : Reshape
  cfblk3 : Delay  DelayLengthSource=Input port  SampleTime=1
      settings: InputPortMap=u0,p1
  cfblk4 : Delay  SampleTime=1
  cfblk5 : simulink/Discrete/Transfer Fcn Real Zero  ZeroZ=0.75  ICPrevInput=0.0  DoSatur=off
  cfblk6 : DiscreteFilter  SampleTime=1
  cfblk7 : DiscreteStateSpace
  cfblk8 : Sum  Inputs=+
  cfblk9 : Sum  Inputs=|++
  cfblk2 : Outport
  wires:
  cfblk13/1 -> cfblk4/1
  cfblk11/1 -> cfblk7/1
  cfblk8/1 -> cfblk6/1
  cfblk9/1 -> cfblk2/1
  cfblk1/1 -> cfblk8/1
  cfblk3/1 -> cfblk9/1
  cfblk10/1 -> cfblk11/1
  cfblk12/1 -> cfblk5/1
  cfblk5/1 -> cfblk9/2
  cfblk4/1 -> cfblk10/1
  cfblk7/1 -> cfblk3/1
  cfblk6/1 -> cfblk3/2

== system model/cfblk58/cfblk8 ==
  cfblk1 : Inport
  cfblk9 : Inport  Port=2
  cfblk10 : Inport  Port=3
  cfblk11 : Inport  Port=4
  cfblk12 : Inport  Port=5
  cfblk13 : Inport  Port=6
  cfblk14 : Inport  Port=7
  cfblk18 : Delay  SampleTime=1
  cfblk3 : DiscreteFilter  SampleTime=1
  cfblk4 : Math  Operator=mod
  cfblk5 : Product  Inputs=*
  cfblk6 : Gain  Gain=[-633989241.522944]
  cfblk7 : Sum  Inputs=+
  cfblk8 : Signum
  cfblk2 : Outport
  cfblk15 : Outport  Port=2
  cfblk16 : Outport  Port=3
  cfblk17 : Outport  Port=4
  wires:
  cfblk1/1 -> cfblk3/1
  cfblk10/1 -> cfblk8/1
  cfblk3/1 -> cfblk6/1
  cfblk9/1 -> cfblk4/1
  cfblk12/1 -> cfblk16/1
  cfblk13/1 -> cfblk17/1
  cfblk7/1 -> cfblk5/1
  cfblk8/1 -> cfblk2/1
  cfblk6/1 -> cfblk15/1
  cfblk4/1 -> cfblk7/1
  cfblk5/1 -> cfblk18/1
  cfblk18/1 -> cfblk4/2

== system model/cfblk58/cfblk9 ==
  cfblk1 : Inport
  cfblk9 : Inport  Port=2
  cfblk10 : Inport  Port=3
  cfblk3 : slpidlib/PID Controller (2DOF)  Controller=PID  Form=Parallel  TimeDomain=Discrete-time  UseExternalTs=off  SampleTime=1  IntegratorMethod=Forward Euler  FilterMethod=Forward Euler  ControllerParametersSource=internal  P=1  I=1  UseKiTs=off  D=0  N=100  UseFilter=on  b=1  c=1  TunerSelectOption=Transfer Function Based (PID Tuner App)  InitialConditionSource=internal  InitialConditionForIntegrator=0  InitialConditionForFilter=0  DifferentiatorICPrevScaledInput=0  ExternalReset=none  TrackingMode=off  Kt=1  LimitOutput=off  SatLimitsSource=internal  UpperSaturationLimit=inf  LowerSaturationLimit=-inf  LinearizeAsGain=off  AntiWindupMode=none  Kb=1  LimitIntegrator=off  UpperIntegratorSaturationLimit=inf  LowerIntegratorSaturationLimit=-inf  POutMin=[]  POutMax=[]  IOutMin=[]  IOutMax=[]  DOutMin=[]  DOutMax=[]  NOutMin=[]  NOutMax=[]  bOutMin=[]  bOutMax=[]  cOutMin=[]  cOutMax=[]  SumOutMin=[]  SumOutMax=[]  SaturationOutMin=[]  SaturationOutMax=[]  PParamMin=[]  PParamMax=[]  IParamMin=[]  IParamMax=[]  DParamMin=[]  DParamMax=[]  NParamMin=[]  NParamMax=[]  bParamMin=[]  bParamMax=[]  cParamMin=[]  cParamMax=[]  KbParamMin=[]  KbParamMax=[]  KtParamMin=[]  KtParamMax=[]  KbOutMin=[]  KbOutMax=[]  KtOutMin=[]  KtOutMax=[]  IntegratorOutMin=[]  IntegratorOutMax=[]  FilterOutMin=[]  FilterOutMax=[]  SumI1OutMin=[]  SumI1OutMax=[]  SumI2OutMin=[]  SumI2OutMax=[]  SumI3OutMin=[]  SumI3OutMax=[]  SumI4OutMin=[]  SumI4OutMax=[]  SumDOutMin=[]  SumDOutMax=[]  Sum1OutMin=[]  Sum1OutMax=[]  Sum2OutMin=[]  Sum2OutMax=[]  Sum3OutMin=[]  Sum3OutMax=[]  DifferentiatorOutMin=[]  DifferentiatorOutMax=[]  FilterDiffOutCoefMin=[]  FilterDiffOutCoefMax=[]  ReciprocalOutMin=[]  ReciprocalOutMax=[]  SumDenOutMin=[]  SumDenOutMax=[]  SumNumOutMin=[]  SumNumOutMax=[]  DivideOutMin=[]  DivideOutMax=[]  UdiffTsProdOutMin=[]  UdiffTsProdOutMax=[]  NTsProdOutMin=[]  NTsProdOutMax=[]  UintegralTsProdOutMin=[]  UintegralTsProdOutMax=[]  UngainTsProdOutMin=[]  UngainTsProdOutMax=[]  ClampingZeroOutDataTypeStr=Inherit: Inherit via back propagation  ClampingZeroOutMin=[]  ClampingZeroOutMax=[]  FilterDenConstantOutDataTypeStr=Inherit: Inherit via back propagation  FilterDenConstantOutMin=[]  FilterDenConstantOutMax=[]  PCopyOutDataTypeStr=Inherit: Inherit via back propagation  PCopyOutMin=[]  PCopyOutMax=[]  NCopyOutDataTypeStr=Inherit: Inherit via back propagation  NCopyOutMin=[]  NCopyOutMax=[]  IntegratorContinuousStateAttributes=''  IntegratorStateMustResolveToSignalObject=off  IntegratorRTWStateStorageClass=Auto  FilterContinuousStateAttributes=''  FilterStateMustResolveToSignalObject=off  FilterRTWStateStorageClass=Auto  ParallelPVariant=InternalParameters  IdealPVariant=Disabled  IVariant=InternalParameters  DVariant=InternalParameters  bVariant=InternalParameters  cVariant=InternalParameters  IntegratorVariant=Discrete  SatVariant=Disabled  AWVariant=Passthrough  PCopyVariant=Disabled  TRVariant=Disabled  FdbkBlocksVariant=Forward  IdealPFdbkVariant=Disabled  SatFdbkVariant=Disabled  DerivativeFilterVariant=ForwardEulerFilter  NVariant=InternalParameters  NCopyVariant=Disabled  FilterICVariant=InternalICsFilter  IntegratorICVariant=InternalICs  ExternalResetVariant=Disabled  TRSumVariant=Passthrough  SumFdbkVariant=Disabled  SumVariant=Sum_PID  TsampFilterVariant=InternalTs  TsampNgainVariant=Passthrough  TsampIntegralVariant=Disabled_SignalSpec  ExternalSaturationOutDataTypeStr=Inherit: Same as second input
      settings: LibrarySourceBlock=simulink/Discrete/Discrete PID Controller (2DOF)
  cfblk4 : DiscreteStateSpace
  cfblk5 : ComplexToRealImag
  cfblk6 : Sqrt
  cfblk7 : Sqrt
  cfblk8 : Constant  Value=[-73162090.597440]  SampleTime=1
  cfblk2 : Outport
  cfblk11 : Outport  Port=2
  wires:
  cfblk3/1 -> cfblk6/1
  cfblk4/1 -> cfblk2/1
  cfblk9/1 -> cfblk4/1
  cfblk1/1 -> cfblk11/1
  cfblk5/1 -> cfblk7/1
  cfblk6/1 -> cfblk5/1
  cfblk10/1 -> cfblk3/1
  cfblk8/1 -> cfblk3/2

== system model/cfblk59/cfblk10 ==
  cfblk1 : Inport
  cfblk11 : Inport  Port=2
  cfblk12 : Inport  Port=3
  cfblk13 : Inport  Port=4
  cfblk14 : Inport  Port=5
  cfblk15 : Inport  Port=6
  cfblk10 : Constant  Value=[-799526649.376795]  SampleTime=1
  cfblk17 : DataTypeConversion  SaturateOnIntegerOverflow=off  RndMeth=Floor
  cfblk3 : simulink/Discrete/Transfer Fcn Lead or Lag  PoleZ=0.95  ZeroZ=0.75  ICPrevOutput=0.0  ICPrevInput=0.0  DoSatur=off
  cfblk4 : UnitDelay  HasFrameUpgradeWarning=on
  cfblk5 : DiscreteStateSpace
  cfblk6 : ComplexToMagnitudeAngle
  cfblk7 : Product
  cfblk8 : Product  Inputs=**
  cfblk9 : Gain  Gain=[-51794296.399981]
  cfblk2 : Outport
  cfblk16 : Outport  Port=2
  wires:
  cfblk1/1 -> cfblk9/1
  cfblk8/1 -> cfblk16/1
  cfblk7/1 -> cfblk5/1
  cfblk12/1 -> cfblk2/1
  cfblk11/1 -> cfblk4/1
  cfblk13/1 -> cfblk8/1
  cfblk4/1 -> cfblk3/1
  cfblk3/1 -> cfblk7/1
  cfblk5/1 -> cfblk8/2
  cfblk9/1 -> cfblk7/2
  cfblk14/1 -> cfblk17/1
  cfblk17/1 -> cfblk6/1

== system model/cfblk59/cfblk11 ==
  cfblk1 : Inport
  cfblk10 : Delay  SampleTime=1
  cfblk11 : Delay  SampleTime=1
  cfblk3 : Rounding
  cfblk4 : Sum  Inputs=+-
  cfblk5 : Assignment  DiagnosticForDimensions=Warning  IndexOptions=Index vector (dialog)  Indices=1  OutputSizes=1
  cfblk6 : simulink/Math Operations/MinMax Running Resettable  Function=min  vinit=0.0
  cfblk7 : Sum  Inputs=--
  cfblk2 : Outport
  cfblk8 : Outport  Port=2
  cfblk9 : Outport  Port=3
  wires:
  cfblk1/1 -> cfblk7/1, cfblk6/1, cfblk9/1
  cfblk4/1 -> cfblk6/2, cfblk10/1
  cfblk6/1 -> cfblk3/1, cfblk11/1
  cfblk3/1 -> cfblk2/1, cfblk8/1
  cfblk7/1 -> cfblk5/1, cfblk5/2
  cfblk5/1 -> cfblk4/2
  cfblk10/1 -> cfblk7/2
  cfblk11/1 -> cfblk4/1

== system model/cfblk59/cfblk12 ==
  cfblk1 : Inport
  cfblk8 : Inport  Port=2
  cfblk3 : DiscreteFir  SampleTime=1
  cfblk4 : simulink/Discrete/Transfer Fcn Lead or Lag  PoleZ=0.95  ZeroZ=0.75  ICPrevOutput=0.0  ICPrevInput=0.0  DoSatur=off
  cfblk5 : Gain  Gain=[902161619.426705]
  cfblk6 : MinMax  Function=max  Inputs=3
  cfblk7 : Constant  Value=[865177994.704862]  SampleTime=1
  cfblk2 : Outport
  wires:
  cfblk7/1 -> cfblk3/1
  cfblk8/1 -> cfblk5/1
  cfblk3/1 -> cfblk2/1
  cfblk1/1 -> cfblk4/1, cfblk6/3
  cfblk4/1 -> cfblk6/1
  cfblk5/1 -> cfblk6/2

== system model/cfblk60/cfblk8 ==
  cfblk1 : Inport
  cfblk9 : Inport  Port=2
  cfblk10 : Inport  Port=3
  cfblk11 : Inport  Port=4
  cfblk12 : Inport  Port=5
  cfblk3 : Delay  DelayLengthSource=Input port  SampleTime=1
      settings: InputPortMap=u0,p1
  cfblk4 : ComplexToMagnitudeAngle
  cfblk5 : Reshape
  cfblk6 : ComplexToRealImag
  cfblk7 : Constant  Value=[102961489.191398]  SampleTime=1
  cfblk8 : Constant  Value=[-890234968.492882]  SampleTime=1
  cfblk2 : Outport
  cfblk13 : Outport  Port=2
  cfblk14 : Outport  Port=3
  wires:
  cfblk10/1 -> cfblk6/1
  cfblk7/1 -> cfblk3/1
  cfblk8/1 -> cfblk5/1
  cfblk4/1 -> cfblk2/1
  cfblk6/1 -> cfblk3/2
  cfblk12/1 -> cfblk14/1
  cfblk9/1 -> cfblk4/1
  cfblk4/2 -> cfblk13/1

== system model/cfblk60/cfblk9 ==
  cfblk1 : Inport
  cfblk10 : Inport  Port=2
  cfblk11 : Inport  Port=3
  cfblk3 : simulink/Discrete/Difference  ICPrevInput=0.0  OutMin=[]  OutMax=[]  OutDataTypeStr=Inherit: Inherit via back propagation  OutDataType=fixdt(1, 16)  OutScaling=2^-10  DoSatur=off
  cfblk4 : simulink/Discrete/Transfer Fcn First Order  PoleZ=0.95  ICPrevOutput=0.0  DoSatur=off
  cfblk5 : Product  Inputs=*
  cfblk6 : Product  Inputs=*
  cfblk7 : Sum  Inputs=|++
  cfblk8 : Constant  Value=[172466346.597371]  SampleTime=1
  cfblk9 : Constant  Value=[-113647376.115251]  SampleTime=1
  cfblk2 : Outport
  wires:
  cfblk5/1 -> cfblk7/1
  cfblk9/1 -> cfblk5/1
  cfblk4/1 -> cfblk2/1
  cfblk1/1 -> cfblk7/2
  cfblk7/1 -> cfblk3/1
  cfblk10/1 -> cfblk4/1
  cfblk8/1 -> cfblk6/1

== system model/cfblk61/cfblk10 ==
  cfblk1 : Inport
  cfblk10 : Inport  Port=2
  cfblk11 : Delay  SampleTime=1
  cfblk3 : slpidlib/PID Controller (2DOF)  Controller=PID  Form=Parallel  TimeDomain=Discrete-time  UseExternalTs=off  SampleTime=1  IntegratorMethod=Forward Euler  FilterMethod=Forward Euler  ControllerParametersSource=internal  P=1  I=1  UseKiTs=off  D=0  N=100  UseFilter=on  b=1  c=1  TunerSelectOption=Transfer Function Based (PID Tuner App)  InitialConditionSource=internal  InitialConditionForIntegrator=0  InitialConditionForFilter=0  DifferentiatorICPrevScaledInput=0  ExternalReset=none  TrackingMode=off  Kt=1  LimitOutput=off  SatLimitsSource=internal  UpperSaturationLimit=inf  LowerSaturationLimit=-inf  LinearizeAsGain=off  AntiWindupMode=none  Kb=1  LimitIntegrator=off  UpperIntegratorSaturationLimit=inf  LowerIntegratorSaturationLimit=-inf  POutMin=[]  POutMax=[]  IOutMin=[]  IOutMax=[]  DOutMin=[]  DOutMax=[]  NOutMin=[]  NOutMax=[]  bOutMin=[]  bOutMax=[]  cOutMin=[]  cOutMax=[]  SumOutMin=[]  SumOutMax=[]  SaturationOutMin=[]  SaturationOutMax=[]  PParamMin=[]  PParamMax=[]  IParamMin=[]  IParamMax=[]  DParamMin=[]  DParamMax=[]  NParamMin=[]  NParamMax=[]  bParamMin=[]  bParamMax=[]  cParamMin=[]  cParamMax=[]  KbParamMin=[]  KbParamMax=[]  KtParamMin=[]  KtParamMax=[]  KbOutMin=[]  KbOutMax=[]  KtOutMin=[]  KtOutMax=[]  IntegratorOutMin=[]  IntegratorOutMax=[]  FilterOutMin=[]  FilterOutMax=[]  SumI1OutMin=[]  SumI1OutMax=[]  SumI2OutMin=[]  SumI2OutMax=[]  SumI3OutMin=[]  SumI3OutMax=[]  SumI4OutMin=[]  SumI4OutMax=[]  SumDOutMin=[]  SumDOutMax=[]  Sum1OutMin=[]  Sum1OutMax=[]  Sum2OutMin=[]  Sum2OutMax=[]  Sum3OutMin=[]  Sum3OutMax=[]  DifferentiatorOutMin=[]  DifferentiatorOutMax=[]  FilterDiffOutCoefMin=[]  FilterDiffOutCoefMax=[]  ReciprocalOutMin=[]  ReciprocalOutMax=[]  SumDenOutMin=[]  SumDenOutMax=[]  SumNumOutMin=[]  SumNumOutMax=[]  DivideOutMin=[]  DivideOutMax=[]  UdiffTsProdOutMin=[]  UdiffTsProdOutMax=[]  NTsProdOutMin=[]  NTsProdOutMax=[]  UintegralTsProdOutMin=[]  UintegralTsProdOutMax=[]  UngainTsProdOutMin=[]  UngainTsProdOutMax=[]  ClampingZeroOutDataTypeStr=Inherit: Inherit via back propagation  ClampingZeroOutMin=[]  ClampingZeroOutMax=[]  FilterDenConstantOutDataTypeStr=Inherit: Inherit via back propagation  FilterDenConstantOutMin=[]  FilterDenConstantOutMax=[]  PCopyOutDataTypeStr=Inherit: Inherit via back propagation  PCopyOutMin=[]  PCopyOutMax=[]  NCopyOutDataTypeStr=Inherit: Inherit via back propagation  NCopyOutMin=[]  NCopyOutMax=[]  IntegratorContinuousStateAttributes=''  IntegratorStateMustResolveToSignalObject=off  IntegratorRTWStateStorageClass=Auto  FilterContinuousStateAttributes=''  FilterStateMustResolveToSignalObject=off  FilterRTWStateStorageClass=Auto  ParallelPVariant=InternalParameters  IdealPVariant=Disabled  IVariant=InternalParameters  DVariant=InternalParameters  bVariant=InternalParameters  cVariant=InternalParameters  IntegratorVariant=Discrete  SatVariant=Disabled  AWVariant=Passthrough  PCopyVariant=Disabled  TRVariant=Disabled  FdbkBlocksVariant=Forward  IdealPFdbkVariant=Disabled  SatFdbkVariant=Disabled  DerivativeFilterVariant=ForwardEulerFilter  NVariant=InternalParameters  NCopyVariant=Disabled  FilterICVariant=InternalICsFilter  IntegratorICVariant=InternalICs  ExternalResetVariant=Disabled  TRSumVariant=Passthrough  SumFdbkVariant=Disabled  SumVariant=Sum_PID  TsampFilterVariant=InternalTs  TsampNgainVariant=Passthrough  TsampIntegralVariant=Disabled_SignalSpec  ExternalSaturationOutDataTypeStr=Inherit: Same as second input
      settings: LibrarySourceBlock=simulink/Discrete/Discrete PID Controller (2DOF)
  cfblk4 : simulink/Discrete/Transfer Fcn Real Zero  ZeroZ=0.75  ICPrevInput=0.0  DoSatur=off
  cfblk5 : DiscreteZeroPole  Poles=[0 0.5]  Gain=1
  cfblk6 : Signum
  cfblk7 : Gain  Gain=[299264373.631218]
  cfblk8 : Constant  Value=[-280929519.369593]  SampleTime=1
  cfblk9 : Constant  Value=[-222455009.243467]  SampleTime=1
  cfblk2 : Outport
  wires:
  cfblk3/1 -> cfblk6/1
  cfblk9/1 -> cfblk5/1
  cfblk5/1 -> cfblk4/1
  cfblk8/1 -> cfblk2/1
  cfblk10/1 -> cfblk7/1
  cfblk1/1 -> cfblk3/2
  cfblk6/1 -> cfblk11/1
  cfblk11/1 -> cfblk3/1

== system model/cfblk61/cfblk11 ==
  cfblk1 : Inport
  cfblk10 : Inport  Port=2
  cfblk11 : Inport  Port=3
  cfblk12 : Inport  Port=4
  cfblk3 : simulink/Discrete/Difference  ICPrevInput=0.0  OutMin=[]  OutMax=[]  OutDataTypeStr=Inherit: Inherit via back propagation  OutDataType=fixdt(1, 16)  OutScaling=2^-10  DoSatur=off
  cfblk4 : simulink/Discrete/Difference  ICPrevInput=0.0  OutMin=[]  OutMax=[]  OutDataTypeStr=Inherit: Inherit via back propagation  OutDataType=fixdt(1, 16)  OutScaling=2^-10  DoSatur=off
  cfblk5 : DotProduct  OutDataTypeStr=Inherit: Inherit via internal rule
  cfblk6 : Sqrt
  cfblk7 : Sum  Inputs=|++
  cfblk8 : Reshape
  cfblk9 : Constant  Value=[-936052059.241793]  SampleTime=1
  cfblk2 : Outport
  cfblk13 : Outport  Port=2
  wires:
  cfblk12/1 -> cfblk3/1
  cfblk7/1 -> cfblk2/1
  cfblk10/1 -> cfblk6/1
  cfblk4/1 -> cfblk13/1
  cfblk1/1 -> cfblk8/1
  cfblk11/1 -> cfblk4/1
  cfblk6/1 -> cfblk7/1
  cfblk9/1 -> cfblk5/1
  cfblk5/1 -> cfblk7/2
  cfblk3/1 -> cfblk5/2

== system model/cfblk61/cfblk12 ==
  cfblk1 : Inport
  cfblk10 : Inport  Port=2
  cfblk11 : Inport  Port=3
  cfblk12 : Delay  SampleTime=1
  cfblk13 : Delay  SampleTime=1
  cfblk3 : simulink/Discrete/Transfer Fcn Real Zero  ZeroZ=0.75  ICPrevInput=0.0  DoSatur=off
  cfblk4 : DiscreteZeroPole  Poles=[0 0.5]  Gain=1
  cfblk5 : Delay  DelayLengthSource=Input port  SampleTime=1
      settings: InputPortMap=u0,p1
  cfblk6 : Bias  Bias=[-410248870.074913]  SaturateOnIntegerOverflow=off
  cfblk7 : PermuteDimensions
  cfblk8 : Sum  Inputs=|++
  cfblk9 : Rounding
  cfblk2 : Outport
  wires:
  cfblk1/1 -> cfblk4/1
  cfblk10/1 -> cfblk3/1
  cfblk7/1 -> cfblk9/1
  cfblk11/1 -> cfblk2/1
  cfblk3/1 -> cfblk8/1
  cfblk6/1 -> cfblk7/1
  cfblk5/1 -> cfblk8/2
  cfblk4/1 -> cfblk5/2
  cfblk8/1 -> cfblk12/1
  cfblk12/1 -> cfblk5/1
  cfblk9/1 -> cfblk13/1
  cfblk13/1 -> cfblk6/1
